simulink model "LED_Example"  (R2022a)
settings: Solver=FixedStepAuto  StartTime=0.0  StopTime=10.0  FixedStep=1e-3  RelTol=1e-3  EnableMultiTasking=on
libraries: frdmk64flib x1
settings Model: ExtModeTrigDuration=5  Creator=ethan  LastModifiedBy=ethan
settings OptimizationCC: EnhancedBackFolding=on  PassReuseOutputArgsAs=Individual arguments  ZeroExternalMemoryAtStartup=off  ZeroInternalMemoryAtStartup=off  MaxStackSize=64  OptimizeBlockOrder=speed  DifferentSizesBufferReuse=on  OptimizationCustomize=off  EfficientTunableParamExpr=on
settings DebuggingCC: ParameterTunabilityLossMsg=error
settings HardwareCC: ProdBitPerPointer=32  ProdBitPerSizeT=32  ProdBitPerPtrDiffT=32  ProdLargestAtomicInteger=Long  ProdLargestAtomicFloat=Double  ProdWordSize=32  ProdHWDeviceType=ARM Compatible->ARM Cortex
settings SFSimCC: MATLABDynamicMemAlloc=off
settings RTWCC: SystemTargetFile=ert.tlc  HardwareBoard=NXP FRDM-K64F  TLCOptions="-aInlineSetEventsForThisBaseRateFcn=TLC_FALSE -aSuppressMultiTaskScheduler=TLC_FALSE  -aRateBasedStepFcn=0"  TemplateMakefile=ert_default_tmf  Toolchain=GNU Tools for ARM Embedded Processors
settings CodeAppCC: ForceParamTrailComments=on  IgnoreCustomStorageClasses=off  OperatorAnnotations=on  SimulinkDataObjDesc=on  SFDataObjDesc=on  InsertBlockDesc=on
settings ERTTargetCC: ExtModeTransport=4  ExtModeMexFile=sendToCommService

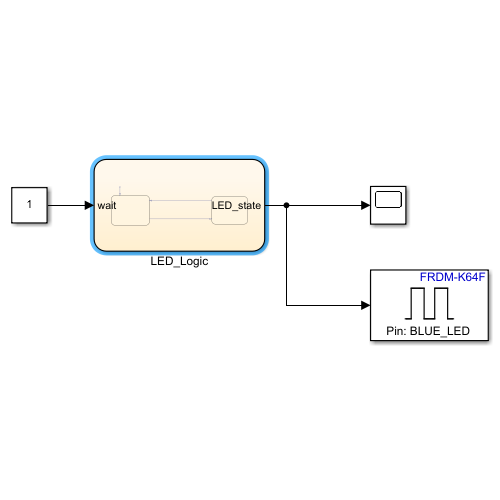
[thumbnail: Simulink's stored preview of the top-level diagram]
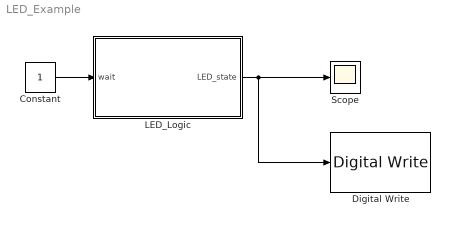
== system LED_Example ==
  Constant : Constant  OutDataTypeStr=int8
  Digital Write : frdmk64flib/Digital Write  Whichpin=BLUE_LED
  LED_Logic : Stateflow chart  TreatAsAtomicUnit=on
  Scope : Scope
  wires:
  Constant/1 -> LED_Logic/1(wait)
  LED_Logic/1(LED_state) -> Scope/1, Digital Write/1

== stateflow chart LED_Example/LED_Logic ==
  state LED_On
    entry:
    LED_state = true;
  state LED_Off
    entry:
    LED_state = false;
  (default) -> LED_On
  LED_Off -> LED_On : after(wait,sec)
  LED_On -> LED_Off : after(1000,msec)
  data: LED_state output boolean; wait input int8
